simulink model "Vehicle_Model_Controller_Sep26"  (R2020b)
settings: Solver=VariableStepAuto  StartTime=0.0  StopTime=60  FixedStep=0.001  RelTol=1e-3
model workspace (MAT data in the model file):
  Kp = 10
  understeer_gradient = 0.05
undefined symbols (not defined in the file or in its folder): front_forces, rear_forces
libraries: fl_lib x24, nesl_utility x20, sdl_lib x8, pid_lib x1, vehdynlibsteering x1, autolibshared x1, autolibdatasheetbattery x1
(part 1 of 2)
settings Model: TunableVars=F_sv,F_x_ij,F_x_ij_max,F_y_fl,F_y_fr,F_y_ij,F_y_rl,F_y_rr,J_z,K_1,K_2,LB,PID,R,T_x_ij,UP,delta,driver_input,err,l,l_f,l_r,linsol,s,s_f,s_r,x,x_1,x_2,x_3,x_4,y,y_1,y_2,y_3,y_4  TunableVarsStorageClass=Auto,Auto,Auto,Auto,Auto,Auto,Auto,Auto,Auto,Auto,Auto,Auto,Auto,Auto,Auto,Auto,Auto,Auto,Auto,Auto,Auto,Auto,Auto,Auto,Auto,Auto,Auto,Auto,Auto,Auto,Auto,Auto,Auto,Auto,Auto,Auto  TunableVarsTypeQualifier=,,,,,,,,,,,,,,,,,,,,,,,,,,,,,,,,,,,  ParameterArgumentNames=understeer_gradient  OrderedModelArguments=off  Creator=True  LastModifiedBy=Inver
settings SolverCC: MinimalZcImpactIntegration=on
settings DataIOCC: ExternalInput=Sheet1.getElement('driver_input'),Sheet1.getElement('P_A'),Sheet1.getElement('steering_angle'),Sheet1.getElement('b_FL'),Sheet1.getElement('b_FR'),Sheet1.getElement('b_RL'),Sheet1.getElement('b_RR'),Sheet1.getElement('wind x'),Sheet1.getElement('wind y'),Sheet1.getElement('wind z'),Sheet1.getElement('batt_temp')  LoadExternalInput=on
settings OptimizationCC: DefaultParameterBehavior=Inlined  GainParamInheritBuiltInType=on  UseFloatMulNetSlope=on  InlineInvariantSignals=on  BufferReuse=off  EnhancedBackFolding=on  PassReuseOutputArgsThreshold=0  EfficientFloat2IntCast=on  EfficientMapNaN2IntZero=off  OptimizeBlockOrder=speed  DifferentSizesBufferReuse=on
settings DebuggingCC: RTPrefix=warning  ReadBeforeWriteMsg=DisableAll  WriteAfterWriteMsg=DisableAll  WriteAfterReadMsg=DisableAll  SolverPrmCheckMsg=error  MultiTaskDSMMsg=none  ParameterTunabilityLossMsg=error  ArithmeticOperatorsInVariantConditions=warning
settings HardwareCC: TargetBitPerPointer=64  TargetBitPerSizeT=64  TargetBitPerPtrDiffT=64  TargetLongLongMode=on  TargetIntDivRoundTo=Zero  TargetEndianess=LittleEndian  TargetWordSize=64  TargetHWDeviceType=MATLAB Host  ProdEqTarget=off
settings ModelReferenceCC: UpdateModelReferenceTargets=IfOutOfDate
settings SFSimCC: SimUserIncludeDirs=$matlabroot$\toolbox\rtw\rtwdemos\EmbeddedCoderOverview\  SFSimEcho=off  SimAnalyzeCustomCode=on  MATLABDynamicMemAlloc=off  CustomCodeUndefinedFunction=UseInterfaceOnly
settings RTWCC: Description=Rapid Simulation Target  SystemTargetFile=rsim.tlc  GenCodeOnly=on  TemplateMakefile=rsim_default_tmf  GenerateReport=on  BuildConfiguration=Faster Runs  LaunchReport=on  CheckMdlBeforeBuild=Warning
settings CodeAppCC: ForceParamTrailComments=on  OperatorAnnotations=on
settings RSimTargetCC: TargetLangStandard=C99 (ISO)
settings ConfigComp: CovScope=ReferencedModels  DVMaxProcessTime=100  DVTestSuiteOptimization=Auto  DVDetectOutOfBounds=on
settings SimscapeCC: SimscapeLogType=local

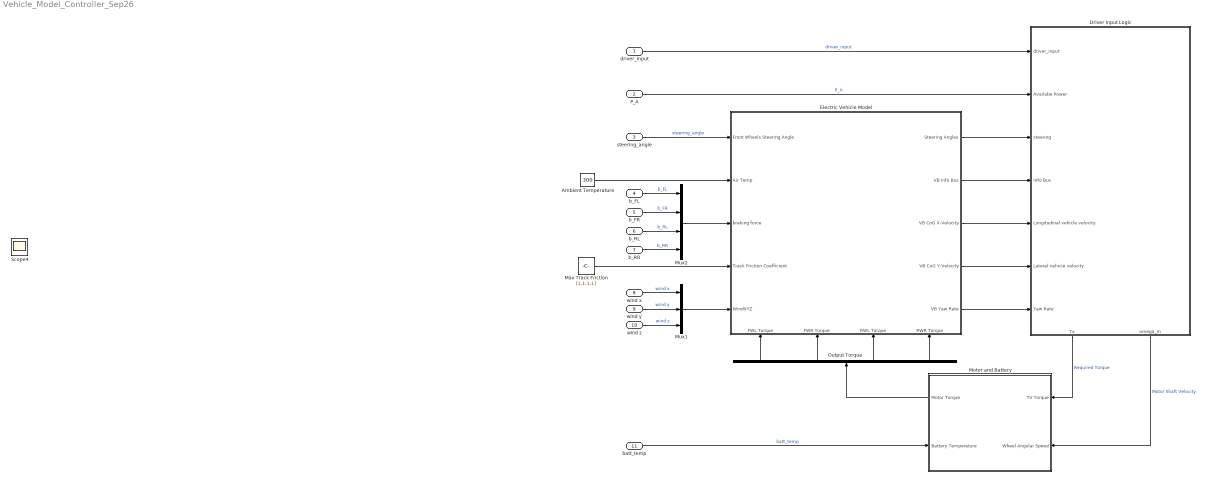
== system Vehicle_Model_Controller_Sep26 ==
  driver_input : Inport  Interpolate=off
  P_A : Inport  Port=2  Interpolate=off
  steering_angle : Inport  Port=3
  b_FL : Inport  Port=4
  b_FR : Inport  Port=5
  b_RL : Inport  Port=6
  b_RR : Inport  Port=7
  wind x : Inport  Port=8
  wind y : Inport  Port=9
  wind z : Inport  Port=10
  batt_temp : Inport  Port=11
  Ambient Temperature : Constant  Value=300
  Driver Input Logic : Subsystem
      settings: PortSchema="{\"entries\":[{\"content\":{\"sides\":[{\"content\":{\"connectorIds\":[\"In1\",\"In2\",\"In3\",\"In4\",\"In5\",\"In6\",\"In7\"]},\"type\":\"ConnectorPlacement.EquallySpacedRectSide\",\"uuid\":\"d4eb2ff2-232d-44db-a8b8-a4c31f4610ca\"},{\"content\":{\"connectorIds\":[],\"side\":\"RIGHT\"},\"type\":\"ConnectorPlacement.EquallySpacedRectSide\",\"uuid\":\"689b9a1f-e3f2-4125-bcde-f52737465846\"},{\"content\":{\"connectorIds\":[],\"side\":\"TOP\"},\"type\":\"ConnectorPlacement.EquallySpacedRectSide\",\"uuid\":\"ac555b84-9566-43e7-b127-ef70ed4803a8\"},{\"content\":{\"connectorIds\":[\"Out1\",\"Out2\"],\"side\":\"BOTTOM\"},\"type\":\"ConnectorPlacement.EquallySpacedRectSide\",\"uuid\":\"c1bd47d4-1445-408b-adbe-f2c4bc464b6e\"},{\"content\":{\"connectorIds\":[],\"side\":\"HIDDEN\"},\"type\":\"ConnectorPlacement.EquallySpacedRectSide\",\"uuid\":\"7b18933c-f262-4964-9433-4f333eec7628\"}]},\"type\":\"ConnectorPlacement.EquallySpacedConnector\",\"uuid\":\"306bffda-2c1f-46fb-8755-5ea28e33f612\"}],\"packageUris\":[\"http://schema.mathworks.com/mf0/Connector/R2020b\"],\"version\":\"1.0\"}"
  Electric Vehicle Model : Subsystem
      settings: PortSchema="{\"entries\":[{\"content\":{\"sides\":[{\"content\":{\"connectorIds\":[\"In1\",\"In2\",\"In3\",\"In4\",\"In5\"]},\"type\":\"ConnectorPlacement.EquallySpacedRectSide\",\"uuid\":\"d116468d-7868-487f-a964-21d40fbcc809\"},{\"content\":{\"connectorIds\":[\"Out1\",\"Out2\",\"Out3\",\"Out4\",\"Out5\"],\"side\":\"RIGHT\"},\"type\":\"ConnectorPlacement.EquallySpacedRectSide\",\"uuid\":\"69901164-3ba1-4787-94a1-b6dad3f5570f\"},{\"content\":{\"connectorIds\":[],\"side\":\"TOP\"},\"type\":\"ConnectorPlacement.EquallySpacedRectSide\",\"uuid\":\"0399aa14-7cbc-406a-a0bc-5234930aa618\"},{\"content\":{\"connectorIds\":[\"In6\",\"In7\",\"In8\",\"In9\"],\"side\":\"BOTTOM\"},\"type\":\"ConnectorPlacement.EquallySpacedRectSide\",\"uuid\":\"c6246111-4a4d-44a6-9f60-6dbbfa6f6be1\"}]},\"type\":\"ConnectorPlacement.EquallySpacedConnector\",\"uuid\":\"33585625-d9f5-41d4-8b4d-b29cb62e09b6\"}],\"packageUris\":[\"http://schema.mathworks.com/mf0/Connector/R2020b\"],\"version\":\"1.0\"}"
  Max Track Friction : Constant  Value=[1,1;1,1]
  Motor and Battery : Subsystem
      settings: PortSchema="{\"entries\":[{\"content\":{\"sides\":[{\"content\":{\"connectorIds\":[\"Out1\",\"In1\"]},\"type\":\"ConnectorPlacement.EquallySpacedRectSide\",\"uuid\":\"d5eb6e01-74de-485f-b814-f74cf87d6300\"},{\"content\":{\"connectorIds\":[\"In2\",\"In3\"],\"side\":\"RIGHT\"},\"type\":\"ConnectorPlacement.EquallySpacedRectSide\",\"uuid\":\"4e9b95b3-1238-4789-a4cc-20b236b4d536\"},{\"content\":{\"connectorIds\":[],\"side\":\"TOP\"},\"type\":\"ConnectorPlacement.EquallySpacedRectSide\",\"uuid\":\"97fc91bc-a36c-43db-88cf-61ba0348fc60\"},{\"content\":{\"connectorIds\":[],\"side\":\"HIDDEN\"},\"type\":\"ConnectorPlacement.EquallySpacedRectSide\",\"uuid\":\"c955884f-22bb-4f22-9982-ff8bef63f64d\"}]},\"type\":\"ConnectorPlacement.EquallySpacedConnector\",\"uuid\":\"927982b2-ec40-42a1-9f55-58bc607d6a22\"}],\"packageUris\":[\"http://schema.mathworks.com/mf0/Connector/R2020b\"],\"version\":\"1.0\"}"
  Mux1 : Mux  Inputs=3
  Mux2 : Mux
  Output Torque : Demux
  Scope4 : Scope
  wires:
  Ambient Temperature/1 -> Electric Vehicle Model/2(Air Temp)
  Electric Vehicle Model/2(VB Info Bus) -> Driver Input Logic/4(Info Bus)
  Electric Vehicle Model/3(VB CoG X-Velocity) -> Driver Input Logic/5(Longitudinal vehicle velocity)
  Electric Vehicle Model/4(VB CoG Y-Velocity) -> Driver Input Logic/6(Lateral vehicle velocity)
  Electric Vehicle Model/5(VB Yaw Rate) -> Driver Input Logic/7(Yaw Rate)
  driver_input/1 -> Driver Input Logic/1(driver_input)  "driver_input"
  Driver Input Logic/1(Tx) -> Motor and Battery/2(TV Torque)  "Required Torque"
  wind x/1 -> Mux1/1  "wind x"
  wind y/1 -> Mux1/2  "wind y"
  wind z/1 -> Mux1/3  "wind z"
  Mux1/1 -> Electric Vehicle Model/5(WindXYZ)
  b_FR/1 -> Mux2/2  "b_FR"
  b_FL/1 -> Mux2/1  "b_FL"
  b_RL/1 -> Mux2/3  "b_RL"
  b_RR/1 -> Mux2/4  "b_RR"
  Mux2/1 -> Electric Vehicle Model/3(braking force)
  batt_temp/1 -> Motor and Battery/1(Battery Temperature)  "batt_temp"
  Motor and Battery/1(Motor Torque) -> Output Torque/1
  P_A/1 -> Driver Input Logic/2(Availabe Power)  "P_A"
  Max Track Friction/1 -> Electric Vehicle Model/4(Track Friction Coefficient)
  Driver Input Logic/2(omega_m) -> Motor and Battery/3(Wheel Angular Speed)  "Motor Shaft Velocity"
  steering_angle/1 -> Electric Vehicle Model/1(Front Wheels Steering Angle)  "steering_angle"
  Electric Vehicle Model/1(Steering Angles) -> Driver Input Logic/3(steering)
  Output Torque/1 -> Electric Vehicle Model/6(FWL Torque)
  Output Torque/2 -> Electric Vehicle Model/7(FWR Torque)
  Output Torque/3 -> Electric Vehicle Model/8(RWL Torque)
  Output Torque/4 -> Electric Vehicle Model/9(RWR Torque)

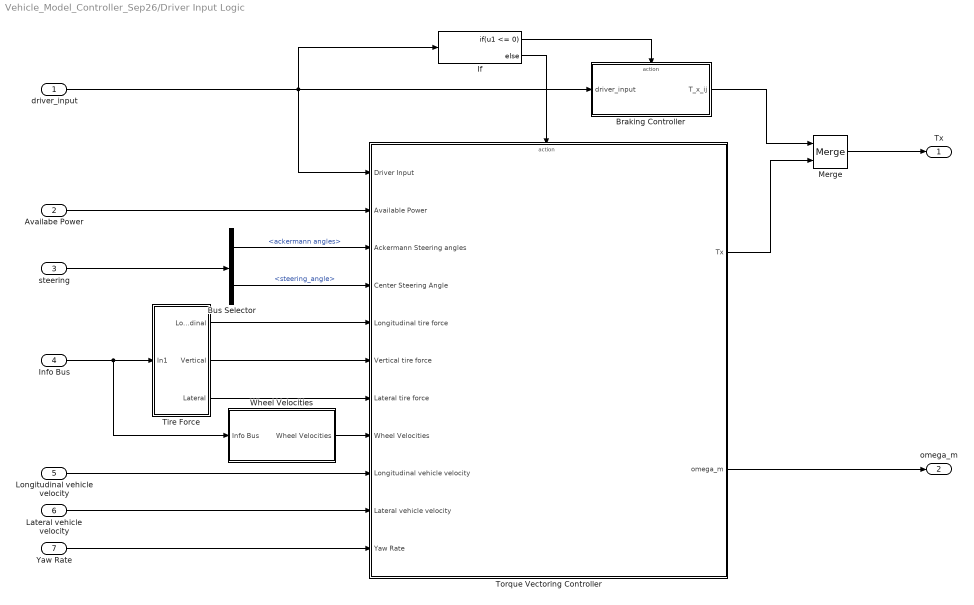
== system Vehicle_Model_Controller_Sep26/Driver Input Logic ==
  driver_input : Inport
  Availabe Power : Inport  Port=2
  steering : Inport  Port=3
  Info Bus : Inport  Port=4
  Longitudinal vehicle velocity : Inport  Port=5
  Lateral vehicle velocity : Inport  Port=6
  Yaw Rate : Inport  Port=7
  Braking Controller : Subsystem
  Bus Selector : BusSelector  OutputSignals=ackermann angles,steering_angle
  If : If  IfExpression=u1 <= 0
  Merge : Merge
  Tire Force : Subsystem
  Torque Vectoring Controller : Subsystem
  Wheel Velocities : Subsystem
  Tx : Outport
  omega_m : Outport  Port=2
  wires:
  Tire Force/1(Longitudinal) -> Torque Vectoring Controller/5(Longitudinal tire force)
  Lateral vehicle velocity/1 -> Torque Vectoring Controller/10(Lateral vehicle velocity)
  Longitudinal vehicle velocity/1 -> Torque Vectoring Controller/9(Longitudinal vehicle velocity)
  Tire Force/2(Vertical) -> Torque Vectoring Controller/6(Vertical tire force)
  Yaw Rate/1 -> Torque Vectoring Controller/11(Yaw Rate)
  If/1 -> Braking Controller/Action
  If/2 -> Torque Vectoring Controller/Action
  Braking Controller/1(T_x_ij) -> Merge/1
  driver_input/1 -> Torque Vectoring Controller/1(Driver Input), Braking Controller/1(driver_input), If/1
  Bus Selector/2 -> Torque Vectoring Controller/4(Center Steering Angle)  "<steering_angle>"
  Tire Force/3(Lateral) -> Torque Vectoring Controller/7(Lateral tire force)
  steering/1 -> Bus Selector/1
  Bus Selector/1 -> Torque Vectoring Controller/3("Ackermann Steering angles ")  "<ackermann angles>"
  Availabe Power/1 -> Torque Vectoring Controller/2(Available Power)
  Info Bus/1 -> Tire Force/1(In1), Wheel Velocities/1(Info Bus)
  Wheel Velocities/1(Wheel Velocities) -> Torque Vectoring Controller/8(Wheel Velocities)
  Merge/1 -> Tx/1
  Torque Vectoring Controller/1(Tx) -> Merge/2
  Torque Vectoring Controller/2(omega_m) -> omega_m/1

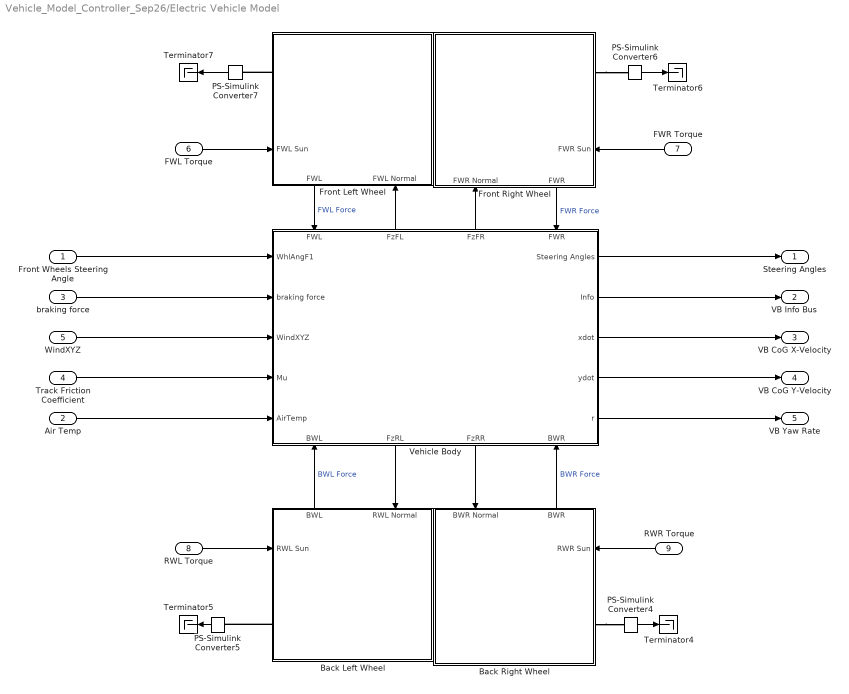
== system Vehicle_Model_Controller_Sep26/Electric Vehicle Model ==
  Front Wheels Steering Angle : Inport
  Air Temp : Inport  Port=2
  braking force : Inport  Port=3
  Track Friction Coefficient : Inport  Port=4
  WindXYZ : Inport  Port=5
  FWL Torque : Inport  Port=6
  FWR Torque : Inport  Port=7
  RWL Torque : Inport  Port=8
  RWR Torque : Inport  Port=9
  Back Left Wheel : Subsystem
      settings: PortSchema="{\"entries\":[{\"content\":{\"sides\":[{\"content\":{\"connectorIds\":[\"In1\",\"LConn1\"]},\"type\":\"ConnectorPlacement.EquallySpacedRectSide\",\"uuid\":\"9f52900f-df3e-41ac-b258-782e5d4e0eaf\"},{\"content\":{\"connectorIds\":[],\"side\":\"RIGHT\"},\"type\":\"ConnectorPlacement.EquallySpacedRectSide\",\"uuid\":\"34c2d9dc-60c7-40ad-be28-599fbc039141\"},{\"content\":{\"connectorIds\":[\"Out1\",\"In2\"],\"side\":\"TOP\"},\"type\":\"ConnectorPlacement.EquallySpacedRectSide\",\"uuid\":\"1dcff801-acc8-4468-b9f1-4bf879f78c2b\"}]},\"type\":\"ConnectorPlacement.EquallySpacedConnector\",\"uuid\":\"fe63b2f8-6027-4789-9c90-5c54dbfc2a0a\"}],\"packageUris\":[\"http://schema.mathworks.com/mf0/Connector/R2020b\"],\"version\":\"1.0\"}"
  Back Right Wheel : Subsystem
      settings: PortSchema="{\"entries\":[{\"content\":{\"sides\":[{\"content\":{\"connectorIds\":[]},\"type\":\"ConnectorPlacement.EquallySpacedRectSide\",\"uuid\":\"9f52900f-df3e-41ac-b258-782e5d4e0eaf\"},{\"content\":{\"connectorIds\":[\"In2\",\"RConn1\"],\"side\":\"RIGHT\"},\"type\":\"ConnectorPlacement.EquallySpacedRectSide\",\"uuid\":\"34c2d9dc-60c7-40ad-be28-599fbc039141\"},{\"content\":{\"connectorIds\":[\"In1\",\"Out1\"],\"side\":\"TOP\"},\"type\":\"ConnectorPlacement.EquallySpacedRectSide\",\"uuid\":\"1dcff801-acc8-4468-b9f1-4bf879f78c2b\"}]},\"type\":\"ConnectorPlacement.EquallySpacedConnector\",\"uuid\":\"fe63b2f8-6027-4789-9c90-5c54dbfc2a0a\"}],\"packageUris\":[\"http://schema.mathworks.com/mf0/Connector/R2020b\"],\"version\":\"1.0\"}"
  Front Left Wheel : Subsystem
      settings: PortSchema="{\"entries\":[{\"content\":{\"sides\":[{\"content\":{\"connectorIds\":[\"LConn1\",\"In1\"]},\"type\":\"ConnectorPlacement.EquallySpacedRectSide\",\"uuid\":\"9f52900f-df3e-41ac-b258-782e5d4e0eaf\"},{\"content\":{\"connectorIds\":[],\"side\":\"RIGHT\"},\"type\":\"ConnectorPlacement.EquallySpacedRectSide\",\"uuid\":\"34c2d9dc-60c7-40ad-be28-599fbc039141\"},{\"content\":{\"connectorIds\":[],\"side\":\"TOP\"},\"type\":\"ConnectorPlacement.EquallySpacedRectSide\",\"uuid\":\"1dcff801-acc8-4468-b9f1-4bf879f78c2b\"},{\"content\":{\"connectorIds\":[\"Out1\",\"In2\"],\"side\":\"BOTTOM\"},\"type\":\"ConnectorPlacement.EquallySpacedRectSide\",\"uuid\":\"4fb396e2-b116-48bf-ae47-9a39d6e53df1\"}]},\"type\":\"ConnectorPlacement.EquallySpacedConnector\",\"uuid\":\"fe63b2f8-6027-4789-9c90-5c54dbfc2a0a\"}],\"packageUris\":[\"http://schema.mathworks.com/mf0/Connector/R2020b\"],\"version\":\"1.0\"}"
  Front Right Wheel : Subsystem
      settings: PortSchema="{\"entries\":[{\"content\":{\"sides\":[{\"content\":{\"connectorIds\":[]},\"type\":\"ConnectorPlacement.EquallySpacedRectSide\",\"uuid\":\"9f52900f-df3e-41ac-b258-782e5d4e0eaf\"},{\"content\":{\"connectorIds\":[\"RConn1\",\"In2\"],\"side\":\"RIGHT\"},\"type\":\"ConnectorPlacement.EquallySpacedRectSide\",\"uuid\":\"34c2d9dc-60c7-40ad-be28-599fbc039141\"},{\"content\":{\"connectorIds\":[],\"side\":\"TOP\"},\"type\":\"ConnectorPlacement.EquallySpacedRectSide\",\"uuid\":\"1dcff801-acc8-4468-b9f1-4bf879f78c2b\"},{\"content\":{\"connectorIds\":[\"In1\",\"Out1\"],\"side\":\"BOTTOM\"},\"type\":\"ConnectorPlacement.EquallySpacedRectSide\",\"uuid\":\"ca39b8f4-a765-4ff2-9936-a2d929862da7\"}]},\"type\":\"ConnectorPlacement.EquallySpacedConnector\",\"uuid\":\"fe63b2f8-6027-4789-9c90-5c54dbfc2a0a\"}],\"packageUris\":[\"http://schema.mathworks.com/mf0/Connector/R2020b\"],\"version\":\"1.0\"}"
  PS-Simulink Converter{4..7} (4 alike) : nesl_utility/PS-Simulink Converter  PhysicalDomain=network_engine_domain  SubClassName=ps_output  LeftPortType=input  RightPortType=output  PseudoPeriodic=off  Frequencies=[]  Unit=inherit  AffineConversion=off
  Terminator{4..7} (4 alike) : Terminator
  Vehicle Body : Subsystem
      settings: PortSchema="{\"entries\":[{\"content\":{\"sides\":[{\"content\":{\"connectorIds\":[\"In1\",\"In2\",\"In3\",\"In4\",\"In5\"]},\"type\":\"ConnectorPlacement.EquallySpacedRectSide\",\"uuid\":\"92155111-f8f4-4af5-b459-626db8603d20\"},{\"content\":{\"connectorIds\":[\"Out1\",\"Out2\",\"Out3\",\"Out4\",\"Out5\"],\"side\":\"RIGHT\"},\"type\":\"ConnectorPlacement.EquallySpacedRectSide\",\"uuid\":\"ae116824-7c15-47a3-8409-e548e47da19f\"},{\"content\":{\"connectorIds\":[\"In6\",\"Out8\",\"Out9\",\"In7\"],\"side\":\"TOP\"},\"type\":\"ConnectorPlacement.EquallySpacedRectSide\",\"uuid\":\"47f131ff-f47a-4e72-9486-74af6f2f1ac7\"},{\"content\":{\"connectorIds\":[\"In8\",\"Out6\",\"Out7\",\"In9\"],\"side\":\"BOTTOM\"},\"type\":\"ConnectorPlacement.EquallySpacedRectSide\",\"uuid\":\"2f2033fb-4ff2-47eb-b510-cc1663364d24\"},{\"content\":{\"connectorIds\":[],\"side\":\"HIDDEN\"},\"type\":\"ConnectorPlacement.EquallySpacedRectSide\",\"uuid\":\"f9b1c4a7-012e-4646-ac9d-ce6bcd7dfdc6\"}]},\"type\":\"ConnectorPlacement.EquallySpacedConnector\",\"uuid\":\"6b8ecd22-cccf-4b6d-aa41-24252124a118\"}],\"packageUris\":[\"http://schema.mathworks.com/mf0/Connector/R2020b\"],\"version\":\"1.0\"}"
  Steering Angles : Outport
  VB Info Bus : Outport  Port=2
  VB CoG X-Velocity : Outport  Port=3
  VB CoG Y-Velocity : Outport  Port=4
  VB Yaw Rate : Outport  Port=5
  wires:
  Vehicle Body/8(FzFL) -> Front Left Wheel/2(FWL Normal)
  RWR Torque/1 -> Back Right Wheel/2(RWR Sun)
  PS-Simulink Converter6/1 -> Terminator6/1
  PS-Simulink Converter5/1 -> Terminator5/1
  Vehicle Body/5(r) -> VB Yaw Rate/1
  PS-Simulink Converter4/1 -> Terminator4/1
  Front Wheels Steering Angle/1 -> Vehicle Body/1(WhlAngF1)
  Back Left Wheel/1(BWL) -> Vehicle Body/8(BWL)  "BWL Force"
  Vehicle Body/6(FzRL) -> Back Left Wheel/2(RWL Normal)
  Back Right Wheel/1(BWR) -> Vehicle Body/9(BWR)  "BWR Force"
  FWL Torque/1 -> Front Left Wheel/1(FWL Sun)
  Vehicle Body/7(FzRR) -> Back Right Wheel/1(BWR Normal)
  Front Right Wheel/1(FWR) -> Vehicle Body/7(FWR)  "FWR Force"
  Air Temp/1 -> Vehicle Body/5(AirTemp)
  braking force/1 -> Vehicle Body/2(braking force)
  WindXYZ/1 -> Vehicle Body/3(WindXYZ)
  Vehicle Body/3(xdot) -> VB CoG X-Velocity/1
  Front Left Wheel/1(FWL) -> Vehicle Body/6(FWL)  "FWL Force"
  Track Friction Coefficient/1 -> Vehicle Body/4(Mu)
  Vehicle Body/2(Info) -> VB Info Bus/1
  FWR Torque/1 -> Front Right Wheel/2(FWR Sun)
  RWL Torque/1 -> Back Left Wheel/1(RWL Sun)
  Vehicle Body/9(FzFR) -> Front Right Wheel/1(FWR Normal)
  PS-Simulink Converter7/1 -> Terminator7/1
  Vehicle Body/4(ydot) -> VB CoG Y-Velocity/1
  Vehicle Body/1(Steering Angles) -> Steering Angles/1
  connections:
  Front Left Wheel/LConn1 -- PS-Simulink Converter7/LConn1
  Back Right Wheel/RConn1 -- PS-Simulink Converter4/LConn1
  Front Right Wheel/RConn1 -- PS-Simulink Converter6/LConn1
  Back Left Wheel/LConn1 -- PS-Simulink Converter5/LConn1

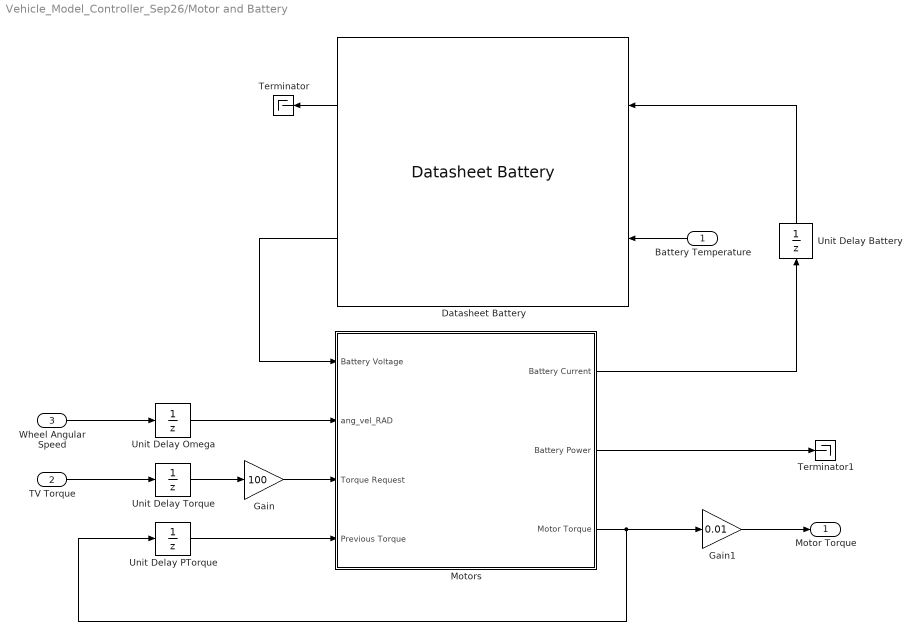
== system Vehicle_Model_Controller_Sep26/Motor and Battery ==
  Battery Temperature : Inport
  TV Torque : Inport  Port=2
  Wheel Angular Speed : Inport  Port=3
  Datasheet Battery : autolibdatasheetbattery/Datasheet Battery  CapacityCtrl=Parameter  OutputVlt=Unfiltered  BattChargeMax=32.5  Em=[2.8 3.228 3.284 3.361 3.408 3.427 3.472 3.477 3.493 3.504 3.516 3.528 3.537 3.545 3.555 3.561 3.566 3.576 3.587 3.589 3.594 3.6 3.608 3.61 3.616 3.619 3.626 3.632 3.637 3.64 3.645 3.646 3.652 3.655 3.658 3.661 3.664 3.668 3.673 3.678 3.68 3.681 3.686 3.692 3.699 3.702 3.705 3.71 3.717 3.723 3.728 3.733 3.735 3.742 3.749 3.755 3.761 3.768 3.773 3.78 3.791 3.798 3.798 3.814 3.818 3.825 3.841 3.846 3.855 3.863 3.877 3.885 3.894 3.907 3.919 3.926 3.935 3.944 3.954 3.964 3.974 3.988 3.998 4.014 4.029 4.034 4.047 4.065 4.074 4.086 4.097 4.131 4.126 4.138 4.15 4.18 4.174 4.187 4.207 4.231 4.221]  CapLUTBp=[0 0.01 0.02 0.03 0.04 0.05 0.06 0.07 0.08 0.09 0.1 0.11 0.12 0.13 0.14 0.15 0.16 0.17 0.18 0.19 0.2 0.21 0.22 0.23 0.24 0.25 0.26 0.27 0.28 0.29 0.3 0.31 0.32 0.33 0.34 0.35 0.36 0.37 0.38 0.39 0.4 0.41 0.42 0.43 0.44 0.45 0.46 0.47 0.48 0.49 0.5 0.51 0.52 0.53 0.54 0.55 0.56 0.57 0.58 0.59 0.6 0.61 0.62 0.63 0.64 0.65 0.66 0.67 0.68 0.69 0.7 0.71 0.72 0.73 0.74 0.75 0.76 0.77 0.78 0.79 0.8 0.81 0.82 0.83 0.84 0.85 0.86 0.87 0.88 0.89 0.9 0.91 0.92 0.93 0.94 0.95 0.96 0.97 0.98 0.99 1]  RInt=[0.008846 0.009319 0.009027 0.00847 0.01032 0.01314;0.006389 0.006554 0.005553 0.005525 0.006043 0.007805;0.004364 0.004101 0.00406 0.003452 0.003846 0.004517;0.002031 0.002563 0.002532 0.00246 0.002716 0.003047;0.001443 0.001825 0.001795 0.001778 0.001924 0.002234;0.0005603 0.0007192 0.0006887 0.0007557 0.0007355 0.001014;0.001028 0.001338 0.001 0.001536 0.001546 0.002789]  BattTempBp=[243.1 253.1 263.1 273.1 283.1 298.1 313.1]  CapSOCBp=[0 0.2 0.4 0.6 0.8 1]  Ns=81  Np=2  BattCapInit=26  Tc=1/1000  Vinit=4.221  RefBlkName='autolibdatasheetbattery/Datasheet Battery'
      settings: SourceProductBaseCode=PW
  Gain : Gain  Gain=100
  Gain1 : Gain  Gain=0.01
  Motors : Subsystem
      mask Display: image('C:\Users\Inver\OneDrive\Desktop\motor.png'); % Use "Edit Image" on toolstrip to change.
  Terminator : Terminator
  Terminator1 : Terminator
  Unit Delay Battery : UnitDelay  SampleTime=-1  HasFrameUpgradeWarning=on
  Unit Delay Omega : UnitDelay  InitialCondition=[0, 0, 0, 0]  SampleTime=-1  HasFrameUpgradeWarning=on
  Unit Delay PTorque : UnitDelay  InitialCondition=[0, 0, 0, 0]  SampleTime=-1  HasFrameUpgradeWarning=on
  Unit Delay Torque : UnitDelay  InitialCondition=[0, 0, 0, 0]  SampleTime=-1  HasFrameUpgradeWarning=on
  Motor Torque : Outport
  wires:
  TV Torque/1 -> Unit Delay Torque/1
  Datasheet Battery/1 -> Terminator/1
  Battery Temperature/1 -> Datasheet Battery/2
  Unit Delay Battery/1 -> Datasheet Battery/1
  Motors/1(Battery Current) -> Unit Delay Battery/1
  Unit Delay Torque/1 -> Gain/1
  Gain/1 -> Motors/3(Torque Request)
  Gain1/1 -> Motor Torque/1
  Motors/3(Motor Torque) -> Unit Delay PTorque/1, Gain1/1
  Motors/2(Battery Power) -> Terminator1/1
  Datasheet Battery/2 -> Motors/1(Battery Voltage)
  Wheel Angular Speed/1 -> Unit Delay Omega/1
  Unit Delay Omega/1 -> Motors/2(ang_vel_RAD)
  Unit Delay PTorque/1 -> Motors/4(Previous Torque)

== system Vehicle_Model_Controller_Sep26/Driver Input Logic/Braking Controller ==
  driver_input : Inport
  Action Port : ActionPort  InitializeStates=reset  PropagateVarSize=During execution  ActionPortLabel=if(u1 <= 0)
  MATLAB Function : MATLAB Function  TreatAsAtomicUnit=on
  T_x_ij : Outport
  wires:
  driver_input/1 -> MATLAB Function/1(driver_input)
  MATLAB Function/1(T_x_ij) -> T_x_ij/1

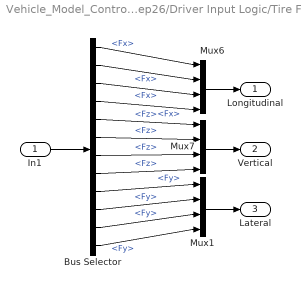
== system Vehicle_Model_Controller_Sep26/Driver Input Logic/Tire Force ==
  In1 : Inport
  Bus Selector : BusSelector  OutputSignals=BdyFrm.Forces.RearAxl.Rght.Fx,BdyFrm.Forces.RearAxl.Lft.Fx,BdyFrm.Forces.FrntAxl.Rght.Fx,BdyFrm.Forces.FrntAxl.Lft.Fx,BdyFrm.Forces.RearAxl.Rght.Fz,BdyFrm.Forces.RearAxl.Lft.Fz,BdyFrm.Forces.FrntAxl.Rght.Fz,BdyFrm.Forces.FrntAxl.Lft.Fz,BdyFrm.Forces.FrntAxl.Lft.Fy,BdyFrm.Forces.FrntAxl.Rght.Fy,BdyFrm.Forces.RearAxl.Lft.Fy,BdyFrm.Forces.RearAxl.Rght.Fy
  Mux1 : Mux
  Mux6 : Mux
  Mux7 : Mux
  Longitudinal : Outport
  Vertical : Outport  Port=2
  Lateral : Outport  Port=3
  wires:
  Bus Selector/2 -> Mux6/2  "<Fx>"
  Bus Selector/8 -> Mux7/4  "<Fz>"
  Bus Selector/5 -> Mux7/1  "<Fz>"
  Bus Selector/6 -> Mux7/2  "<Fz>"
  Bus Selector/1 -> Mux6/1  "<Fx>"
  Mux6/1 -> Longitudinal/1
  Bus Selector/4 -> Mux6/4  "<Fx>"
  Bus Selector/3 -> Mux6/3  "<Fx>"
  Bus Selector/7 -> Mux7/3  "<Fz>"
  Mux7/1 -> Vertical/1
  In1/1 -> Bus Selector/1
  Mux1/1 -> Lateral/1
  Bus Selector/9 -> Mux1/1  "<Fy>"
  Bus Selector/10 -> Mux1/2  "<Fy>"
  Bus Selector/11 -> Mux1/3  "<Fy>"
  Bus Selector/12 -> Mux1/4  "<Fy>"

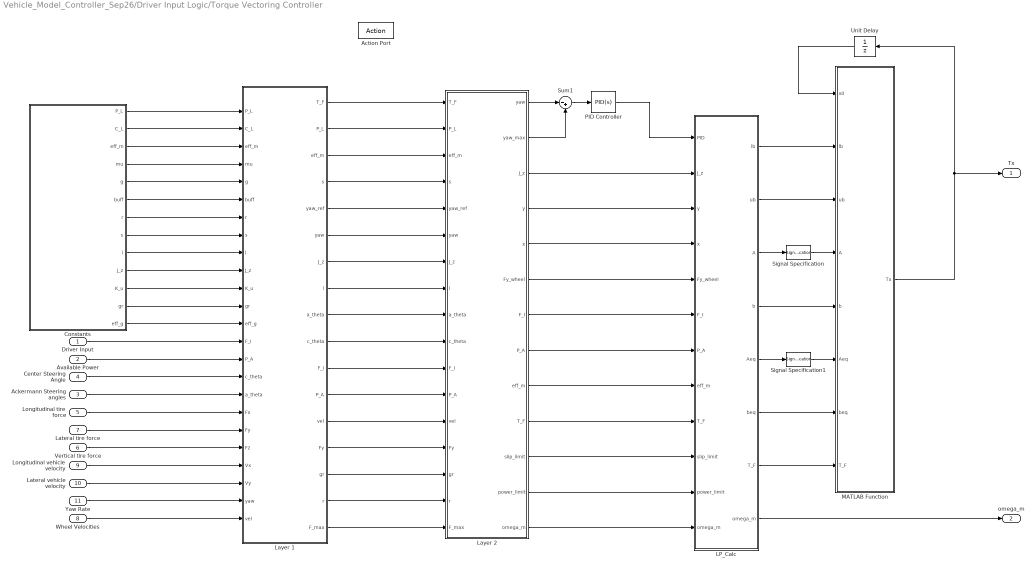
== system Vehicle_Model_Controller_Sep26/Driver Input Logic/Torque Vectoring Controller ==
  Driver Input : Inport
  Available Power : Inport  Port=2
  "Ackermann Steering angles " : Inport  Port=3
  Center Steering Angle : Inport  Port=4
  Longitudinal tire force : Inport  Port=5
  Vertical tire force : Inport  Port=6
  Lateral tire force : Inport  Port=7
  Wheel Velocities : Inport  Port=8
  Longitudinal vehicle velocity : Inport  Port=9
  Lateral vehicle velocity : Inport  Port=10
  Yaw Rate : Inport  Port=11
  Action Port : ActionPort  InitializeStates=reset  PropagateVarSize=During execution  ActionPortLabel=else
  "Constants " : MATLAB Function  TreatAsAtomicUnit=on
  "LP_Calc " : MATLAB Function
  Layer 1 : MATLAB Function  TreatAsAtomicUnit=on
  Layer 2 : MATLAB Function  TreatAsAtomicUnit=on
  MATLAB Function : MATLAB Function
  PID Controller : pid_lib/PID Controller  Controller=PID  Form=Parallel  TimeDomain=Continuous-time  UseExternalTs=off  SampleTime=-1  IntegratorMethod=Forward Euler  FilterMethod=Forward Euler  ControllerParametersSource=internal  P=40  I=3  D=0  UseFilter=on  N=100  TunerSelectOption=Transfer Function Based (PID Tuner App)  InitialConditionSource=internal  InitialConditionForIntegrator=0  InitialConditionForFilter=0  DifferentiatorICPrevScaledInput=0  ExternalReset=none  TrackingMode=off  Kt=1  LimitOutput=on  SatLimitsSource=internal  UpperSaturationLimit=inf  LowerSaturationLimit=-inf  LinearizeAsGain=on  AntiWindupMode=back-calculation  Kb=1  POutMin=[]  POutMax=[]  IOutMin=[]  IOutMax=[]  DOutMin=[]  DOutMax=[]  NOutMin=[]  NOutMax=[]  SumOutMin=[]  SumOutMax=[]  SaturationOutMin=[]  SaturationOutMax=[]  PParamMin=[]  PParamMax=[]  IParamMin=[]  IParamMax=[]  DParamMin=[]  DParamMax=[]  NParamMin=[]  NParamMax=[]  KbParamMin=[]  KbParamMax=[]  KtParamMin=[]  KtParamMax=[]  KbOutMin=[]  KbOutMax=[]  KtOutMin=[]  KtOutMax=[]  IntegratorOutMin=[]  IntegratorOutMax=[]  FilterOutMin=[]  FilterOutMax=[]  SumI1OutMin=[]  SumI1OutMax=[]  SumI2OutMin=[]  SumI2OutMax=[]  SumI3OutMin=[]  SumI3OutMax=[]  SumI4OutMin=[]  SumI4OutMax=[]  SumDOutMin=[]  SumDOutMax=[]  DifferentiatorOutMin=[]  DifferentiatorOutMax=[]  FilterDiffOutCoefMin=[]  FilterDiffOutCoefMax=[]  ReciprocalOutMin=[]  ReciprocalOutMax=[]  SumDenOutMin=[]  SumDenOutMax=[]  SumNumOutMin=[]  SumNumOutMax=[]  DivideOutMin=[]  DivideOutMax=[]  UdiffTsProdOutMin=[]  UdiffTsProdOutMax=[]  NTsProdOutMin=[]  NTsProdOutMax=[]  UintegralTsProdOutMin=[]  UintegralTsProdOutMax=[]  UngainTsProdOutMin=[]  UngainTsProdOutMax=[]  IntegratorContinuousStateAttributes=''  IntegratorStateMustResolveToSignalObject=off  IntegratorRTWStateStorageClass=Auto  FilterContinuousStateAttributes=''  FilterStateMustResolveToSignalObject=off  FilterRTWStateStorageClass=Auto  ParallelPVariant=InternalParameters  IdealPVariant=Disabled  IVariant=InternalParameters  DVariant=InternalParameters  IntegratorVariant=Continuous  SatVariant=Enabled  AWVariant=BackCalculation  PCopyVariant=Disabled  TRVariant=Disabled  FdbkBlocksVariant=Forward  IdealPFdbkVariant=Disabled  SatFdbkVariant=Disabled  DerivativeFilterVariant=ContFilter  NVariant=InternalParameters  NCopyVariant=Disabled  FilterICVariant=InternalICsFilter  IntegratorICVariant=InternalICs  ExternalResetVariant=Disabled  TRSumVariant=Passthrough  SumFdbkVariant=Disabled  SumVariant=Sum_PID  TsampFilterVariant=InternalTs  TsampNgainVariant=Passthrough  TsampIntegralVariant=Passthrough  ExternalSaturationOutDataTypeStr=Inherit: Same as second input
  Signal Specification : SignalSpecification  Dimensions=[1 4]
  Signal Specification1 : SignalSpecification  Dimensions=[1 4]
  Sum1 : Sum  Inputs=|-+
  Unit Delay : UnitDelay  InitialCondition=[0, 0, 0, 0]  SampleTime=-1  HasFrameUpgradeWarning=on
  Tx : Outport
  omega_m : Outport  Port=2
  wires:
  "Constants "/2(C_L) -> Layer 1/2(C_L)
  Driver Input/1 -> Layer 1/14("F_I ")
  "Constants "/13(eff_g) -> Layer 1/13(eff_g)
  Layer 1/1(T_F) -> Layer 2/1("T_F ")
  Longitudinal tire force/1 -> Layer 1/18(Fx)
  Sum1/1 -> PID Controller/1
  Layer 1/8(l) -> Layer 2/8(l)
  Layer 2/12(power_limit) -> "LP_Calc "/11(power_limit)
  "Constants "/7(r) -> Layer 1/7("r ")
  "Constants "/9(l) -> Layer 1/9("l ")
  Layer 1/16(r) -> Layer 2/16(r)
  Available Power/1 -> Layer 1/15("P_A ")
  Yaw Rate/1 -> Layer 1/23("yaw ")
  Layer 1/10(c_theta) -> Layer 2/10(c_theta)
  Layer 1/9(a_theta) -> Layer 2/9(a_theta)
  Layer 1/13(vel) -> Layer 2/13(vel)
  "Constants "/3(eff_m) -> Layer 1/3("eff_m ")
  Layer 2/5(x) -> "LP_Calc "/4(x)
  Layer 1/3(eff_m) -> Layer 2/3("eff_m ")
  Layer 2/11(slip_limit) -> "LP_Calc "/10(slip_limit)
  Layer 2/2(yaw_max) -> Sum1/2
  "Constants "/11(K_u) -> Layer 1/11(K_u)
  Layer 1/17(F_max) -> Layer 2/17(F_max)
  "Constants "/5(g) -> Layer 1/5(g)
  Layer 1/14(Fy) -> Layer 2/14(Fy)
  "Constants "/1(P_L) -> Layer 1/1("P_L ")
  Longitudinal vehicle velocity/1 -> Layer 1/21(Vx)
  Layer 2/1(yaw) -> Sum1/1
  Layer 2/9(eff_m) -> "LP_Calc "/8(eff_m)
  "Constants "/6(buff) -> Layer 1/6(buff)
  Layer 1/15(gr) -> Layer 2/15(gr)
  Layer 1/2(P_L) -> Layer 2/2(P_L)
  "Ackermann Steering angles "/1 -> Layer 1/17("a_theta ")
  Lateral vehicle velocity/1 -> Layer 1/22(Vy)
  Layer 2/8(P_A) -> "LP_Calc "/7(P_A)
  Center Steering Angle/1 -> Layer 1/16("c_theta ")
  Wheel Velocities/1 -> Layer 1/24("vel ")
  "Constants "/10(J_z) -> Layer 1/10("J_z ")
  Layer 1/5(yaw_ref) -> Layer 2/5(yaw_ref)
  Vertical tire force/1 -> Layer 1/20(Fz)
  "Constants "/4(mu) -> Layer 1/4(mu)
  Lateral tire force/1 -> Layer 1/19("Fy ")
  Layer 2/4(y) -> "LP_Calc "/3(y)
  PID Controller/1 -> "LP_Calc "/1(PID)
  "Constants "/8(s) -> Layer 1/8("s ")
  Layer 2/3(J_z) -> "LP_Calc "/2(J_z)
  Layer 1/4(s) -> Layer 2/4(s)
  "Constants "/12(gr) -> Layer 1/12("gr ")
  Layer 2/7(F_I) -> "LP_Calc "/6(F_I)
  Layer 2/6(Fy_wheel) -> "LP_Calc "/5(Fy_wheel)
  Layer 1/6(yaw) -> Layer 2/6("yaw ")
  Layer 1/7(J_z) -> Layer 2/7("J_z ")
  Layer 1/11(F_I) -> Layer 2/11("F_I ")
  Layer 1/12(P_A) -> Layer 2/12("P_A ")
  Layer 2/10(T_F) -> "LP_Calc "/9("T_F ")
  Layer 2/13(omega_m) -> "LP_Calc "/12("omega_m ")
  Unit Delay/1 -> MATLAB Function/1(x0)
  "LP_Calc "/1(lb) -> MATLAB Function/2(lb)
  "LP_Calc "/2(ub) -> MATLAB Function/3(ub)
  MATLAB Function/1(Tx) -> Unit Delay/1, Tx/1
  "LP_Calc "/4(b) -> MATLAB Function/5(b)
  "LP_Calc "/6(beq) -> MATLAB Function/7(beq)
  "LP_Calc "/8(omega_m) -> omega_m/1
  "LP_Calc "/7(T_F) -> MATLAB Function/8(T_F)
  Signal Specification/1 -> MATLAB Function/4(A)
  "LP_Calc "/3(A) -> Signal Specification/1
  Signal Specification1/1 -> MATLAB Function/6(Aeq)
  "LP_Calc "/5(Aeq) -> Signal Specification1/1

== system Vehicle_Model_Controller_Sep26/Driver Input Logic/Wheel Velocities ==
  Info Bus : Inport
  Bus Selector1 : BusSelector  OutputSignals=BdyFrm.FrntAxl.Lft.Vel.xdot,BdyFrm.FrntAxl.Lft.Vel.ydot,BdyFrm.FrntAxl.Rght.Vel.xdot,BdyFrm.FrntAxl.Rght.Vel.ydot,BdyFrm.RearAxl.Lft.Vel.xdot,BdyFrm.RearAxl.Rght.Vel.xdot
  Mux : Mux  Inputs=6
  Wheel Velocities : Outport
  wires:
  Bus Selector1/3 -> Mux/3  "<xdot>"
  Bus Selector1/2 -> Mux/2  "<ydot>"
  Info Bus/1 -> Bus Selector1/1
  Bus Selector1/6 -> Mux/6  "<xdot>"
  Bus Selector1/4 -> Mux/4  "<ydot>"
  Bus Selector1/1 -> Mux/1  "<xdot>"
  Bus Selector1/5 -> Mux/5  "<xdot>"
  Mux/1 -> Wheel Velocities/1

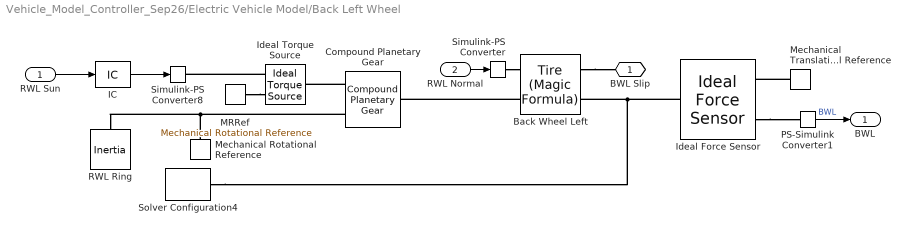
== system Vehicle_Model_Controller_Sep26/Electric Vehicle Model/Back Left Wheel ==
  RWL Sun : Inport
  RWL Normal : Inport  Port=2
  Back Wheel Left : sdl_lib/Tires & Vehicles/Tire (Magic Formula)  parameterization=sdl.enum.magic_tire_model.peak  F_z1=3000 N  F_x1=3500 N  kappa1=10  B_m=10  C_m=1.9  D_m=1  E_m=0.97  fz0=4000 N  p_Cx=1.685  p_Dx=[1.21, -.037]  p_Ex=[.344, .095, -.02, 0]  p_Kx=[21.51, -.163, .245]  p_Hx=[-.002, .002]  p_Vx=[0, 0]  v_tr_thr=0.1 m/s  r_e=0.3 m  model_compliance=0  stiffness=1e6 N/m  damping=1000 N/(m/s)  model_inertia=0  inertia=1 kg*m^2  initial_velocity=0 rad/s  model_resistance=0  resistance_model=1  coeff=0.015  p_tire=250e3 Pa  alpha=-0.003  beta=0.97  coeff_a=84e-4  coeff_b=6.2e-4 s/m  coeff_c=1.6e-4 s^2/m^2  v_thr=0.001 m/s
  Compound Planetary Gear : sdl_lib/Gears/Compound Planetary Gear  rp_ratio=84/23  ps_ratio=40/21  friction_model=sdl.enum.gear_friction.none  mu_visc=[0, 0] N*m/(rad/s)  efficiency=[.96, .98]  temperature_TLU=[280, 300, 320] K  efficiency_sp_TLU=[.95, .9, .85]  efficiency_rp_TLU=[.95, .9, .85]  pwr_thr=[.001, .001] W  thermal_mass=50 J/K  T_init=300 K  model_inertia=simscape.enum.onoff.off  planet_inertia=0.001 kg*m^2
      settings: SourceProductBaseCode=LD  InternalSimscapePortConfiguration="{\"Bottom\":[],\"Left\":[{\"id\":\"C\",\"label\":\"C\",\"type\":\"foundation.mechanical.rotational.rotational\"}],\"Right\":[{\"id\":\"R\",\"label\":\"R\",\"type\":\"foundation.mechanical.rotational.rotational\"},{\"id\":\"S\",\"label\":\"S\",\"type\":\"foundation.mechanical.rotational.rotational\"}],\"Top\":[]}"
  IC : InitialCondition  Value=0
  Ideal Force Sensor : fl_lib/Mechanical/Mechanical Sensors/Ideal Force Sensor
  Ideal Torque Source : fl_lib/Mechanical/Mechanical Sources/Ideal Torque Source
      settings: SourceProductName=Foundation Library
  MRRef : fl_lib/Mechanical/Rotational Elements/Mechanical Rotational Reference
      settings: SourceProductName=Foundation Library
  Mechanical Rotational Reference : fl_lib/Mechanical/Rotational Elements/Mechanical Rotational Reference
  Mechanical Translational Reference : fl_lib/Mechanical/Translational Elements/Mechanical Translational Reference
  PS-Simulink Converter1 : nesl_utility/PS-Simulink Converter  PhysicalDomain=network_engine_domain  SubClassName=ps_output  LeftPortType=input  RightPortType=output  PseudoPeriodic=off  Frequencies=[]  Unit=N  AffineConversion=off
      settings: SourceProductBaseCode=PW,SS
  RWL Ring : fl_lib/Mechanical/Rotational Elements/Inertia  inertia=0.1 kg*m^2  num_ports=foundation.enum.numPorts2.one  w_specify=off  w_priority=High  w=0 rad/s  w_nominal_specify=off  w_nominal_unit=rad/s  w_nominal_value=1  t_specify=off  t_priority=None  t=0 N*m  t_nominal_specify=off  t_nominal_unit=N*m  t_nominal_value=1
  Simulink-PS Converter : nesl_utility/Simulink-PS Converter  PhysicalDomain=network_engine_domain  SubClassName=ps_input  LeftPortType=input  RightPortType=output  PseudoPeriodic=off  Frequencies=[]  NoiseDistribution=none  NoiseParameters=[]  Unit=N  AffineConversion=off  FilteringAndDerivatives=zero  SimscapeFilterOrder=1  InputFilterTimeConstant=0.001  UdotUserProvided=0
      settings: SourceProductBaseCode=PW,SS
  Simulink-PS Converter8 : nesl_utility/Simulink-PS Converter  PhysicalDomain=network_engine_domain  SubClassName=ps_input  LeftPortType=input  RightPortType=output  PseudoPeriodic=off  Frequencies=[]  NoiseDistribution=none  NoiseParameters=[]  Unit=N*m  AffineConversion=off  FilteringAndDerivatives=zero  SimscapeFilterOrder=1  InputFilterTimeConstant=0.001  UdotUserProvided=0
      settings: SourceProductBaseCode=PW,SS
  Solver Configuration4 : nesl_utility/Solver Configuration  PhysicalDomain=network_engine_domain  SubClassName=solver  LeftPortType=input  RightPortType=generic  Tones=[]  Harmonics=[]  SimulateNoise=off  Profile=off  UseLocalSampling=off  EnableSwitchedLinearOptims=on  FrequencyDomain=off  UseCCode=off  RelTol=0.001  AbsTol=1e-06  MinStep=1e-09  ToWorkspace=off  RevertToSquareIcSolve=off  NumHomotopyIterations=100  PhasorMode=off  PhasorModeNumHarmonics=1  DoDC=on  ResidualTolerance=1e-09  UseLocalSolver=off  LocalSolverChoice=NE_BACKWARD_EULER_ADVANCER  LocalSolverSampleTime=0.001  DoFixedCost=off  MaxNonlinIter=3  MaxModeIter=2  ComputeImpulses=off  ImpulseIterations=2  LinearAlgebra=auto  EquationFormulation=NE_TIME_EF  DelaysMemoryBudget=1024  AutomaticFiltering=on  FilteringTimeConstant=0.001  PartitionStorageMethod=AS_NEEDED  PartitionMemoryBudget=1024  PartitionMethod=ROBUST
      settings: SourceProductBaseCode=PW,SS
  BWL Slip : PMIOPort  Side=Left
  BWL : Outport
  wires:
  PS-Simulink Converter1/1 -> BWL/1  "BWL"
  RWL Normal/1 -> Simulink-PS Converter/1
  IC/1 -> Simulink-PS Converter8/1
  RWL Sun/1 -> IC/1
  connections:
  Back Wheel Left/RConn1 -- BWL Slip/RConn1
  Back Wheel Left/LConn2 -- Compound Planetary Gear/LConn1
  Ideal Force Sensor/RConn2 -- PS-Simulink Converter1/LConn1
  Ideal Force Sensor/LConn1 -- Solver Configuration4/RConn1 -- Back Wheel Left/RConn2
  Simulink-PS Converter/RConn1 -- Back Wheel Left/LConn1
  Mechanical Translational Reference/LConn1 -- Ideal Force Sensor/RConn1
  Mechanical Rotational Reference/LConn1 -- RWL Ring/LConn1 -- Compound Planetary Gear/RConn1
  Ideal Torque Source/RConn1 -- Simulink-PS Converter8/RConn1
  Compound Planetary Gear/RConn2 -- Ideal Torque Source/LConn1
  MRRef/LConn1 -- Ideal Torque Source/RConn2

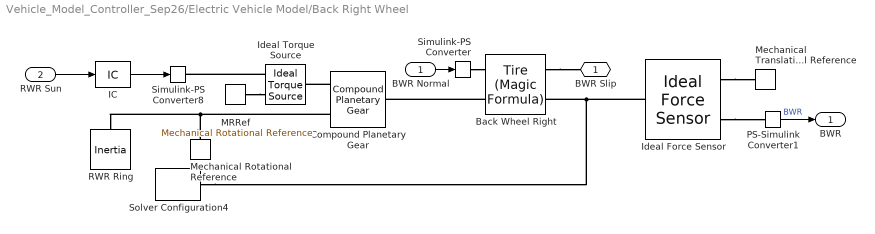
== system Vehicle_Model_Controller_Sep26/Electric Vehicle Model/Back Right Wheel ==
  BWR Normal : Inport
  RWR Sun : Inport  Port=2
  Back Wheel Right : sdl_lib/Tires & Vehicles/Tire (Magic Formula)  parameterization=sdl.enum.magic_tire_model.peak  F_z1=3000 N  F_x1=3500 N  kappa1=10  B_m=10  C_m=1.9  D_m=1  E_m=0.97  fz0=4000 N  p_Cx=1.685  p_Dx=[1.21, -.037]  p_Ex=[.344, .095, -.02, 0]  p_Kx=[21.51, -.163, .245]  p_Hx=[-.002, .002]  p_Vx=[0, 0]  v_tr_thr=0.1 m/s  r_e=0.3 m  model_compliance=0  stiffness=1e6 N/m  damping=1000 N/(m/s)  model_inertia=0  inertia=1 kg*m^2  initial_velocity=0 rad/s  model_resistance=0  resistance_model=1  coeff=0.015  p_tire=250e3 Pa  alpha=-0.003  beta=0.97  coeff_a=84e-4  coeff_b=6.2e-4 s/m  coeff_c=1.6e-4 s^2/m^2  v_thr=0.001 m/s
  Compound Planetary Gear : sdl_lib/Gears/Compound Planetary Gear  rp_ratio=84/23  ps_ratio=40/21  friction_model=sdl.enum.gear_friction.none  mu_visc=[0, 0] N*m/(rad/s)  efficiency=[.96, .98]  temperature_TLU=[280, 300, 320] K  efficiency_sp_TLU=[.95, .9, .85]  efficiency_rp_TLU=[.95, .9, .85]  pwr_thr=[.001, .001] W  thermal_mass=50 J/K  T_init=300 K  model_inertia=simscape.enum.onoff.off  planet_inertia=0.001 kg*m^2
      settings: SourceProductBaseCode=LD  InternalSimscapePortConfiguration="{\"Bottom\":[],\"Left\":[{\"id\":\"C\",\"label\":\"C\",\"type\":\"foundation.mechanical.rotational.rotational\"}],\"Right\":[{\"id\":\"R\",\"label\":\"R\",\"type\":\"foundation.mechanical.rotational.rotational\"},{\"id\":\"S\",\"label\":\"S\",\"type\":\"foundation.mechanical.rotational.rotational\"}],\"Top\":[]}"
  IC : InitialCondition  Value=0
  Ideal Force Sensor : fl_lib/Mechanical/Mechanical Sensors/Ideal Force Sensor
  Ideal Torque Source : fl_lib/Mechanical/Mechanical Sources/Ideal Torque Source
      settings: SourceProductName=Foundation Library
  MRRef : fl_lib/Mechanical/Rotational Elements/Mechanical Rotational Reference
      settings: SourceProductName=Foundation Library
  Mechanical Rotational Reference : fl_lib/Mechanical/Rotational Elements/Mechanical Rotational Reference
  Mechanical Translational Reference : fl_lib/Mechanical/Translational Elements/Mechanical Translational Reference
  PS-Simulink Converter1 : nesl_utility/PS-Simulink Converter  PhysicalDomain=network_engine_domain  SubClassName=ps_output  LeftPortType=input  RightPortType=output  PseudoPeriodic=off  Frequencies=[]  Unit=inherit  AffineConversion=off
      settings: SourceProductBaseCode=PW,SS
  RWR Ring : fl_lib/Mechanical/Rotational Elements/Inertia  inertia=0.1 kg*m^2  num_ports=foundation.enum.numPorts2.one  w_specify=off  w_priority=High  w=0 rad/s  w_nominal_specify=off  w_nominal_unit=rad/s  w_nominal_value=1  t_specify=off  t_priority=None  t=0 N*m  t_nominal_specify=off  t_nominal_unit=N*m  t_nominal_value=1
  Simulink-PS Converter : nesl_utility/Simulink-PS Converter  PhysicalDomain=network_engine_domain  SubClassName=ps_input  LeftPortType=input  RightPortType=output  PseudoPeriodic=off  Frequencies=[]  NoiseDistribution=none  NoiseParameters=[]  Unit=N  AffineConversion=off  FilteringAndDerivatives=zero  SimscapeFilterOrder=1  InputFilterTimeConstant=0.001  UdotUserProvided=0
      settings: SourceProductBaseCode=PW,SS
  Simulink-PS Converter8 : nesl_utility/Simulink-PS Converter  PhysicalDomain=network_engine_domain  SubClassName=ps_input  LeftPortType=input  RightPortType=output  PseudoPeriodic=off  Frequencies=[]  NoiseDistribution=none  NoiseParameters=[]  Unit=N*m  AffineConversion=off  FilteringAndDerivatives=zero  SimscapeFilterOrder=1  InputFilterTimeConstant=0.001  UdotUserProvided=0
      settings: SourceProductBaseCode=PW,SS
  Solver Configuration4 : nesl_utility/Solver Configuration  PhysicalDomain=network_engine_domain  SubClassName=solver  LeftPortType=input  RightPortType=generic  Tones=[]  Harmonics=[]  SimulateNoise=off  Profile=off  UseLocalSampling=off  EnableSwitchedLinearOptims=on  FrequencyDomain=off  UseCCode=off  RelTol=0.001  AbsTol=1e-06  MinStep=1e-09  ToWorkspace=off  RevertToSquareIcSolve=off  NumHomotopyIterations=100  PhasorMode=off  PhasorModeNumHarmonics=1  DoDC=on  ResidualTolerance=1e-09  UseLocalSolver=off  LocalSolverChoice=NE_BACKWARD_EULER_ADVANCER  LocalSolverSampleTime=0.001  DoFixedCost=off  MaxNonlinIter=3  MaxModeIter=2  ComputeImpulses=off  ImpulseIterations=2  LinearAlgebra=auto  EquationFormulation=NE_TIME_EF  DelaysMemoryBudget=1024  AutomaticFiltering=on  FilteringTimeConstant=0.001  PartitionStorageMethod=AS_NEEDED  PartitionMemoryBudget=1024  PartitionMethod=ROBUST
      settings: SourceProductBaseCode=PW,SS
  BWR Slip : PMIOPort  Side=Right
  BWR : Outport
  wires:
  PS-Simulink Converter1/1 -> BWR/1  "BWR"
  BWR Normal/1 -> Simulink-PS Converter/1
  IC/1 -> Simulink-PS Converter8/1
  RWR Sun/1 -> IC/1
  connections:
  Back Wheel Right/RConn1 -- BWR Slip/RConn1
  Ideal Force Sensor/RConn2 -- PS-Simulink Converter1/LConn1
  Ideal Force Sensor/LConn1 -- Solver Configuration4/RConn1 -- Back Wheel Right/RConn2
  Simulink-PS Converter/RConn1 -- Back Wheel Right/LConn1
  Ideal Force Sensor/RConn1 -- Mechanical Translational Reference/LConn1
  Back Wheel Right/LConn2 -- Compound Planetary Gear/LConn1
  Mechanical Rotational Reference/LConn1 -- RWR Ring/LConn1 -- Compound Planetary Gear/RConn1
  Ideal Torque Source/RConn1 -- Simulink-PS Converter8/RConn1
  Compound Planetary Gear/RConn2 -- Ideal Torque Source/LConn1
  MRRef/LConn1 -- Ideal Torque Source/RConn2

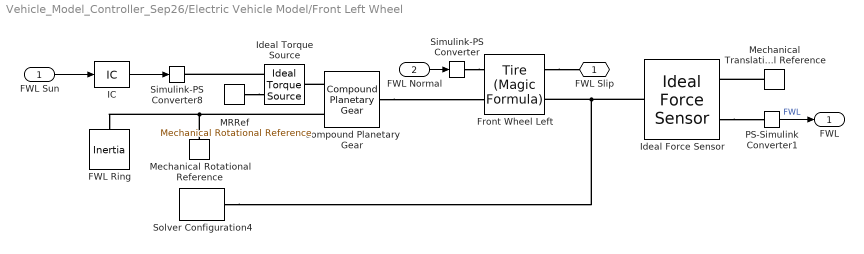
== system Vehicle_Model_Controller_Sep26/Electric Vehicle Model/Front Left Wheel ==
  FWL Sun : Inport
  FWL Normal : Inport  Port=2
  Compound Planetary Gear : sdl_lib/Gears/Compound Planetary Gear  rp_ratio=84/23  ps_ratio=37/24  friction_model=sdl.enum.gear_friction.none  mu_visc=[0, 0] N*m/(rad/s)  efficiency=[.96, .98]  temperature_TLU=[280, 300, 320] K  efficiency_sp_TLU=[.95, .9, .85]  efficiency_rp_TLU=[.95, .9, .85]  pwr_thr=[.001, .001] W  thermal_mass=50 J/K  T_init=300 K  model_inertia=simscape.enum.onoff.off  planet_inertia=0.001 kg*m^2
      settings: SourceProductBaseCode=LD  InternalSimscapePortConfiguration="{\"Bottom\":[],\"Left\":[{\"id\":\"C\",\"label\":\"C\",\"type\":\"foundation.mechanical.rotational.rotational\"}],\"Right\":[{\"id\":\"R\",\"label\":\"R\",\"type\":\"foundation.mechanical.rotational.rotational\"},{\"id\":\"S\",\"label\":\"S\",\"type\":\"foundation.mechanical.rotational.rotational\"}],\"Top\":[]}"
  FWL Ring : fl_lib/Mechanical/Rotational Elements/Inertia  inertia=0.1 kg*m^2  num_ports=foundation.enum.numPorts2.one  w_specify=off  w_priority=High  w=0 rad/s  w_nominal_specify=off  w_nominal_unit=rad/s  w_nominal_value=1  t_specify=off  t_priority=None  t=0 N*m  t_nominal_specify=off  t_nominal_unit=N*m  t_nominal_value=1
  Front Wheel Left : sdl_lib/Tires & Vehicles/Tire (Magic Formula)  parameterization=sdl.enum.magic_tire_model.peak  F_z1=3000 N  F_x1=3500 N  kappa1=10  B_m=10  C_m=1.9  D_m=1  E_m=0.97  fz0=4000 N  p_Cx=1.685  p_Dx=[1.21, -.037]  p_Ex=[.344, .095, -.02, 0]  p_Kx=[21.51, -.163, .245]  p_Hx=[-.002, .002]  p_Vx=[0, 0]  v_tr_thr=0.1 m/s  r_e=0.3 m  model_compliance=0  stiffness=1e6 N/m  damping=1000 N/(m/s)  model_inertia=0  inertia=1 kg*m^2  initial_velocity=0 rad/s  model_resistance=0  resistance_model=1  coeff=0.015  p_tire=250e3 Pa  alpha=-0.003  beta=0.97  coeff_a=84e-4  coeff_b=6.2e-4 s/m  coeff_c=1.6e-4 s^2/m^2  v_thr=0.001 m/s
  IC : InitialCondition  Value=0
  Ideal Force Sensor : fl_lib/Mechanical/Mechanical Sensors/Ideal Force Sensor
  Ideal Torque Source : fl_lib/Mechanical/Mechanical Sources/Ideal Torque Source
      settings: SourceProductName=Foundation Library
  MRRef : fl_lib/Mechanical/Rotational Elements/Mechanical Rotational Reference
      settings: SourceProductName=Foundation Library
  Mechanical Rotational Reference : fl_lib/Mechanical/Rotational Elements/Mechanical Rotational Reference
  Mechanical Translational Reference : fl_lib/Mechanical/Translational Elements/Mechanical Translational Reference
  PS-Simulink Converter1 : nesl_utility/PS-Simulink Converter  PhysicalDomain=network_engine_domain  SubClassName=ps_output  LeftPortType=input  RightPortType=output  PseudoPeriodic=off  Frequencies=[]  Unit=inherit  AffineConversion=off
      settings: SourceProductBaseCode=PW,SS
  Simulink-PS Converter : nesl_utility/Simulink-PS Converter  PhysicalDomain=network_engine_domain  SubClassName=ps_input  LeftPortType=input  RightPortType=output  PseudoPeriodic=off  Frequencies=[]  NoiseDistribution=none  NoiseParameters=[]  Unit=N  AffineConversion=off  FilteringAndDerivatives=zero  SimscapeFilterOrder=1  InputFilterTimeConstant=0.001  UdotUserProvided=0
      settings: SourceProductBaseCode=PW,SS
  Simulink-PS Converter8 : nesl_utility/Simulink-PS Converter  PhysicalDomain=network_engine_domain  SubClassName=ps_input  LeftPortType=input  RightPortType=output  PseudoPeriodic=off  Frequencies=[]  NoiseDistribution=none  NoiseParameters=[]  Unit=N*m  AffineConversion=off  FilteringAndDerivatives=zero  SimscapeFilterOrder=1  InputFilterTimeConstant=0.001  UdotUserProvided=0
      settings: SourceProductBaseCode=PW,SS
  Solver Configuration4 : nesl_utility/Solver Configuration  PhysicalDomain=network_engine_domain  SubClassName=solver  LeftPortType=input  RightPortType=generic  Tones=[]  Harmonics=[]  SimulateNoise=off  Profile=off  UseLocalSampling=off  EnableSwitchedLinearOptims=on  FrequencyDomain=off  UseCCode=off  RelTol=0.001  AbsTol=1e-06  MinStep=1e-09  ToWorkspace=off  RevertToSquareIcSolve=off  NumHomotopyIterations=100  PhasorMode=off  PhasorModeNumHarmonics=1  DoDC=on  ResidualTolerance=1e-09  UseLocalSolver=off  LocalSolverChoice=NE_BACKWARD_EULER_ADVANCER  LocalSolverSampleTime=0.001  DoFixedCost=off  MaxNonlinIter=3  MaxModeIter=2  ComputeImpulses=off  ImpulseIterations=2  LinearAlgebra=auto  EquationFormulation=NE_TIME_EF  DelaysMemoryBudget=1024  AutomaticFiltering=on  FilteringTimeConstant=0.001  PartitionStorageMethod=AS_NEEDED  PartitionMemoryBudget=1024  PartitionMethod=ROBUST
      settings: SourceProductBaseCode=PW,SS
  FWL Slip : PMIOPort  Side=Left
  FWL : Outport
  wires:
  PS-Simulink Converter1/1 -> FWL/1  "FWL"
  FWL Normal/1 -> Simulink-PS Converter/1
  IC/1 -> Simulink-PS Converter8/1
  FWL Sun/1 -> IC/1
  connections:
  Front Wheel Left/RConn1 -- FWL Slip/RConn1
  Compound Planetary Gear/LConn1 -- Front Wheel Left/LConn2
  Ideal Force Sensor/RConn2 -- PS-Simulink Converter1/LConn1
  Ideal Force Sensor/LConn1 -- Solver Configuration4/RConn1 -- Front Wheel Left/RConn2
  Simulink-PS Converter/RConn1 -- Front Wheel Left/LConn1
  Mechanical Translational Reference/LConn1 -- Ideal Force Sensor/RConn1
  Mechanical Rotational Reference/LConn1 -- FWL Ring/LConn1 -- Compound Planetary Gear/RConn1
  Ideal Torque Source/RConn1 -- Simulink-PS Converter8/RConn1
  Compound Planetary Gear/RConn2 -- Ideal Torque Source/LConn1
  MRRef/LConn1 -- Ideal Torque Source/RConn2
